simulink model "simulation"  (R2024b)
settings: Solver=VariableStepAuto  StartTime=0.0  StopTime=15  RelTol=1e-3
libraries: spsMosfetLib x6, simulink x5, spsAsynchronousMachineSIUnitsLib x1, spsDCVoltageSourceLib x1, slpidlib x1, spsThreePhaseVIMeasurementLib x1, spspowerguiLib x1
settings Model: Creator=Yassine  LastModifiedBy=Yassine
settings RTWCC: GPUComputeCapability=3.5

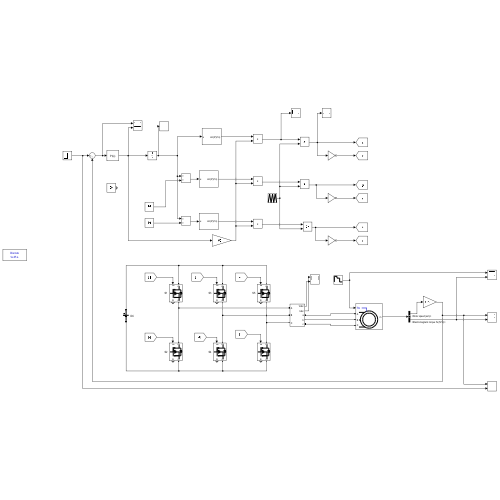
[thumbnail: Simulink's stored preview of the top-level diagram]
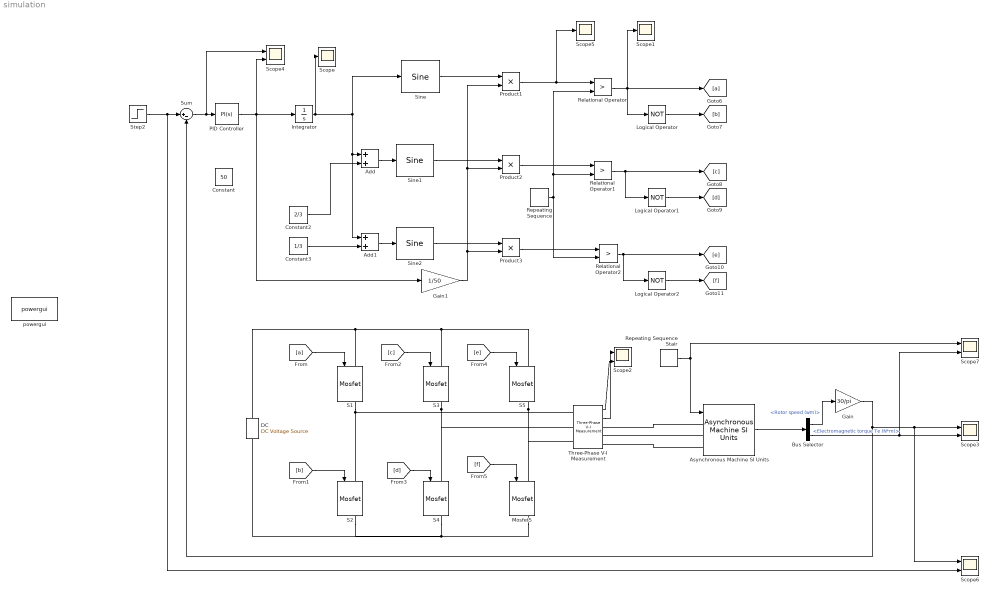
== system simulation ==
  Add : Sum
  Add1 : Sum
  Asynchronous Machine SI Units : spsAsynchronousMachineSIUnitsLib/Asynchronous Machine SI Units  RotorType=Squirrel-cage  PresetModel="15:  5.4 HP (4KW)   400 V  50Hz 1430 RPM"  MechanicalLoad=Torque Tm  ShowDetailedParameters=on  ReferenceFrame=Rotor  Units=SI  MeasurementBus=off  NominalParameters=[4000 400 50]  VoltageRatio=1  Stator=[1.405 0.005839]  Rotor=[1.395 0.005839]  Cage1=[0.4155 0.002066]  Cage2=[0.4168 0.0003495]  Lm=0.1722  Mechanical=[0.0131 0.002985 2]  PolePairs=2  InitialConditions=[0 0 0 0 0 0 0 0]  SimulateSaturation=off  Saturation=[14.03593122, 27.81365428, 53.79336849, 72.68890987, 97.98006896, 148.6815601, 215.7428561, 302.9841135, 428.7778367 ; 230, 322, 414, 460, 506, 552, 598, 644, 690]  LoadFlowParameters=1492000  TsPowergui=0  TsBlock=-1  IterativeModel=Trapezoidal non iterative  IterativeDiscreteModel=Trapezoidal non iterative  Pmec=1.492e+006
  Bus Selector : BusSelector  OutputSignals=Mechanical.Rotor speed (wm),Mechanical.Electromagnetic torque Te (N*m)
  Constant : Constant  Value=50
  Constant2 : Constant  Value=2/3
  Constant3 : Constant  Value=1/3
  DC : spsDCVoltageSourceLib/DC Voltage Source  Amplitude=500  Measurements=None
  Gain : Gain  Gain=30/pi
  Gain1 : Gain  Gain=1/50
  Integrator : Integrator
  Logical Operator : Logic  Operator=NOT  IconShape=distinctive  AllPortsSameDT=off  OutDataTypeStr=boolean
  Logical Operator1 : Logic  Operator=NOT  IconShape=distinctive  AllPortsSameDT=off  OutDataTypeStr=boolean
  Logical Operator2 : Logic  Operator=NOT  IconShape=distinctive  AllPortsSameDT=off  OutDataTypeStr=boolean
  Mosfet5 : spsMosfetLib/Mosfet  Ron=0.1  Lon=0  Rd=0.01  Vfd=0  IC=0  Rs=1e5  Cs=inf  Measurements=on
  PID Controller : slpidlib/PID Controller  Controller=PI  Form=Parallel  TimeDomain=Continuous-time  UseExternalTs=off  SampleTime=-1  IntegratorMethod=Forward Euler  FilterMethod=Forward Euler  ControllerParametersSource=internal  P=.02  I=.5  UseKiTs=off  D=0  UseExternalDerivativeSource=off  N=100  UseFilter=on  TunerSelectOption=Transfer Function Based (PID Tuner App)  InitialConditionSource=internal  InitialConditionForIntegrator=0  InitialConditionForFilter=0  DifferentiatorICPrevScaledInput=0  ExternalReset=none  TrackingMode=off  Kt=1  LimitOutput=off  SatLimitsSource=internal  UpperSaturationLimit=inf  LowerSaturationLimit=-inf  LinearizeAsGain=on  AntiWindupMode=none  Kb=1  LimitIntegrator=off  UpperIntegratorSaturationLimit=inf  LowerIntegratorSaturationLimit=-inf  POutMin=[]  POutMax=[]  IOutMin=[]  IOutMax=[]  DOutMin=[]  DOutMax=[]  NOutMin=[]  NOutMax=[]  SumOutMin=[]  SumOutMax=[]  SaturationOutMin=[]  SaturationOutMax=[]  PParamMin=[]  PParamMax=[]  IParamMin=[]  IParamMax=[]  DParamMin=[]  DParamMax=[]  NParamMin=[]  NParamMax=[]  KbParamMin=[]  KbParamMax=[]  KtParamMin=[]  KtParamMax=[]  KbOutMin=[]  KbOutMax=[]  KtOutMin=[]  KtOutMax=[]  IntegratorOutMin=[]  IntegratorOutMax=[]  FilterOutMin=[]  FilterOutMax=[]  SumI1OutMin=[]  SumI1OutMax=[]  SumI2OutMin=[]  SumI2OutMax=[]  SumI3OutMin=[]  SumI3OutMax=[]  SumI4OutMin=[]  SumI4OutMax=[]  SumDOutMin=[]  SumDOutMax=[]  DifferentiatorOutMin=[]  DifferentiatorOutMax=[]  FilterDiffOutCoefMin=[]  FilterDiffOutCoefMax=[]  ReciprocalOutMin=[]  ReciprocalOutMax=[]  SumDenOutMin=[]  SumDenOutMax=[]  SumNumOutMin=[]  SumNumOutMax=[]  DivideOutMin=[]  DivideOutMax=[]  UdiffTsProdOutMin=[]  UdiffTsProdOutMax=[]  NTsProdOutMin=[]  NTsProdOutMax=[]  UintegralTsProdOutMin=[]  UintegralTsProdOutMax=[]  UngainTsProdOutMin=[]  UngainTsProdOutMax=[]  ClampingZeroOutDataTypeStr=Inherit: Inherit via back propagation  ClampingZeroOutMin=[]  ClampingZeroOutMax=[]  FilterDenConstantOutDataTypeStr=Inherit: Inherit via back propagation  FilterDenConstantOutMin=[]  FilterDenConstantOutMax=[]  PCopyOutDataTypeStr=Inherit: Inherit via back propagation  PCopyOutMin=[]  PCopyOutMax=[]  NCopyOutDataTypeStr=Inherit: Inherit via back propagation  NCopyOutMin=[]  NCopyOutMax=[]  IntegratorContinuousStateAttributes=''  IntegratorStateMustResolveToSignalObject=off  IntegratorRTWStateStorageClass=Auto  FilterContinuousStateAttributes=''  FilterStateMustResolveToSignalObject=off  FilterRTWStateStorageClass=Auto  ParallelPVariant=InternalParameters  IdealPVariant=Disabled  IVariant=InternalParameters  DVariant=Disabled  IntegratorVariant=Continuous  SatVariant=Disabled  AWVariant=Passthrough  PCopyVariant=Disabled  TRVariant=Disabled  FdbkBlocksVariant=Forward  IdealPFdbkVariant=Disabled  SatFdbkVariant=Disabled  DerivativeFilterVariant=Disabled  NVariant=Disabled  NCopyVariant=Disabled_SignalSpec  FilterICVariant=Disabled  IntegratorICVariant=InternalICs  ExternalResetVariant=Disabled  TRSumVariant=Passthrough  SumFdbkVariant=Disabled  SumVariant=Sum_PI  TsampFilterVariant=InternalTs  TsampNgainVariant=Passthrough  TsampIntegralVariant=Disabled_SignalSpec  ExternalSaturationOutDataTypeStr=Inherit: Same as second input  DerivativeSourceVariant=Disabled  PreIntVariant=InternalPreInt
  Product1 : Product
  Product2 : Product
  Product3 : Product
  Relational Operator : RelationalOperator  Operator=>  OutDataTypeStr=boolean  InputSameDT=off
  Relational Operator1 : RelationalOperator  Operator=>  OutDataTypeStr=boolean  InputSameDT=off
  Relational Operator2 : RelationalOperator  Operator=>  OutDataTypeStr=boolean  InputSameDT=off
  Repeating Sequence : simulink/Sources/Repeating Sequence  rep_seq_t=[0 0.5/5000 1/5000]  rep_seq_y=[-1 1 -1]
  Repeating Sequence Stair : simulink/Sources/Repeating Sequence Stair  OutValues=[20 17 10 ]  tsamp=3  OutMin=[]  OutMax=[]  OutDataTypeStr=double  OutputDataTypeScalingMode=double  OutDataType=fixdt(0,8)  ConRadixGroup=Best Precision: Vector-wise  OutScaling=2^-12
  S{1..5} (5 alike) : spsMosfetLib/Mosfet  Ron=0.1  Lon=0  Rd=0.01  Vfd=0  IC=0  Rs=1e5  Cs=inf  Measurements=on
  Scope : Scope
  Scope1 : Scope
  Scope{2..4,6..7} (5 alike) : Scope  NumInputPorts=2
  Scope5 : Scope
  Sine : simulink/Lookup Tables/Sine  Formula=sin(2*pi*u)  NumDataPoints=(2^5)+1  OutputWordLength=16  InternalRulePriority=Speed
  Sine1 : simulink/Lookup Tables/Sine  Formula=sin(2*pi*u)  NumDataPoints=(2^5)+1  OutputWordLength=16  InternalRulePriority=Speed
  Sine2 : simulink/Lookup Tables/Sine  Formula=sin(2*pi*u)  NumDataPoints=(2^5)+1  OutputWordLength=16  InternalRulePriority=Speed
  Step2 : Step  Time=0  Before=1300  After=1430  SampleTime=0
  Sum : Sum  Inputs=|+-
  Three-Phase V-I Measurement : spsThreePhaseVIMeasurementLib/Three-Phase V-I Measurement  VoltageMeasurement=phase-to-phase  SetLabelV=off  LabelV=Vabc  Vpu=off  VpuLL=off  CurrentMeasurement=yes  SetLabelI=off  LabelI=Iabc  Ipu=off  Pbase=100e6  Vbase=500e3  OutputType=Complex  PhasorSimulation=off  PSBequivalent=0
  powergui : spspowerguiLib/powergui  Priority=1  SimulationMode=Discrete  SampleTime=10e-6  frequency=60  Iterations=50  frequencyindice=50  Pbase=100e6  ErrMax=1e-4  UnitsV=kV  UnitsW=MW  buscounter=0  FunctionMessages=off  echomessages=off  EnableUseOfTLC=off  CurrentSourceSwitches=on  DisableSnubberDevices=off  DisableRonSwitches=off  DisableVfSwitches=off  DisplayEquations=off  AutomaticDiscreteSolvers=off  SolverType=Tustin/Backward Euler (TBE)  Interpol=off  ExternalGateDelay=off  methode=off  Ts=100  x0status=blocks  SPID=off  SwTol=0  HookPort=off  NonlinearTolerance=1e-4  nMaxIteration=100  ContinueOnMaxIteration=off  RestoreLinks=warning  ResistiveCurrentMeasurement=off  Frange=[0:2:500]  Ylog=off  Xlog=on  ShowGrid=off  save=off  variable=ZData  structure=0  ZoomFFT=off  StartTime=0.0  cycles=1  DisplayStyle=1  fundamental=60  FreqAxis=off  MaxFrequency=1000  frequencyindicesteady=1  RmsSteady=1  display=off
  wires:
  Logical Operator1/1 -> [d]
  Integrator/1 -> Sine/1, Add1/1, Add/1, Scope/1
  Constant2/1 -> Add/2
  Add1/1 -> Sine2/1
  Constant3/1 -> Add1/2
  Product1/1 -> Scope5/1, Relational Operator/1
  Logical Operator/1 -> [b]
  Logical Operator2/1 -> [f]
  Repeating Sequence/1 -> Relational Operator/2, Relational Operator1/2, Relational Operator2/2
  Sum/1 -> Scope4/1, PID Controller/1
  Three-Phase V-I Measurement/2 -> Scope2/1
  Relational Operator/1 -> Logical Operator/1, [a], Scope1/1
  Bus Selector/2 -> Scope7/2, Scope3/2  "<Electromagnetic torque Te (N*m)>"
  Add/1 -> Sine1/1
  [a] -> S1/1
  Three-Phase V-I Measurement/1 -> Scope2/2
  Gain/1 -> Scope6/1, Scope3/1, Sum/2
  Relational Operator2/1 -> [e], Logical Operator2/1
  [b] -> S2/1
  Relational Operator1/1 -> Logical Operator1/1, [c]
  [c] -> S3/1
  [f] -> Mosfet5/1
  [d] -> S4/1
  Bus Selector/1 -> Gain/1  "<Rotor speed (wm)>"
  Product2/1 -> Relational Operator1/1
  Step2/1 -> Scope6/2, Sum/1
  [e] -> S5/1
  Asynchronous Machine SI Units/1 -> Bus Selector/1
  Repeating Sequence Stair/1 -> Asynchronous Machine SI Units/1, Scope7/1
  Product3/1 -> Relational Operator2/1
  Sine/1 -> Product1/1
  Sine1/1 -> Product2/1
  Sine2/1 -> Product3/1
  Gain1/1 -> Product1/2, Product2/2, Product3/2
  PID Controller/1 -> Gain1/1, Integrator/1, Scope4/2
  connections:
  S1/LConn1 -- DC/RConn1 -- S5/LConn1 -- S3/LConn1
  Three-Phase V-I Measurement/LConn1 -- S1/RConn1 -- S2/LConn1
  S5/RConn1 -- Mosfet5/LConn1 -- Three-Phase V-I Measurement/LConn3
  S3/RConn1 -- S4/LConn1 -- Three-Phase V-I Measurement/LConn2
  S4/RConn1 -- Mosfet5/RConn1 -- DC/LConn1 -- S2/RConn1
  Asynchronous Machine SI Units/LConn1 -- Three-Phase V-I Measurement/RConn1
  Asynchronous Machine SI Units/LConn2 -- Three-Phase V-I Measurement/RConn2
  Asynchronous Machine SI Units/LConn3 -- Three-Phase V-I Measurement/RConn3
